simulink model "HMT_Controller_Testing"  (R2022b)
settings: Solver=VariableStepAuto  StartTime=0.0  StopTime=30.0  RelTol=1e-3
libraries: simulink x1
settings Model: Creator=david  LastModifiedBy=david

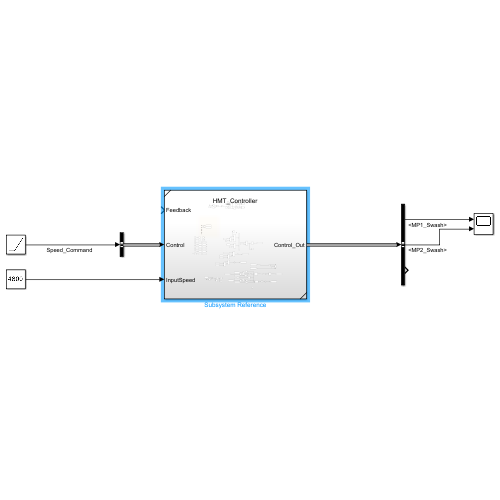
[thumbnail: Simulink's stored preview of the top-level diagram]
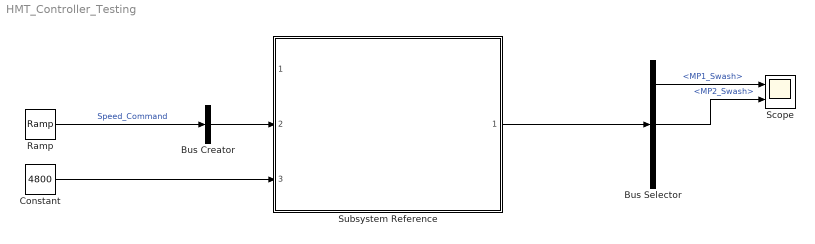
== system HMT_Controller_Testing ==
  Bus Creator : BusCreator  Inputs=1
  Bus Selector : BusSelector  OutputSignals=MP1_Swash,MP2_Swash,Engine_Speed_CMD
  Constant : Constant  Value=4800
  Ramp : simulink/Sources/Ramp  slope=100  start=0  InitialOutput=0
  Scope : Scope  NumInputPorts=2
  Subsystem Reference : Subsystem  ReferencedSubsystem=HMT_Controller
  wires:
  Bus Creator/1 -> Subsystem Reference/2
  Ramp/1 -> Bus Creator/1  "Speed_Command"
  Constant/1 -> Subsystem Reference/3
  Subsystem Reference/1 -> Bus Selector/1
  Bus Selector/1 -> Scope/1  "<MP1_Swash>"
  Bus Selector/2 -> Scope/2  "<MP2_Swash>"
